simulink library "stopSim_ul"  (R2020a)
settings: Solver=VariableStepAuto  StartTime=0.0  StopTime=10.0  RelTol=1e-3
libraries: simulink x2
settings Model: Creator=John Jr  LastModifiedBy=John Jr
settings SFSimCC: CustomCodeUndefinedFunction=UseInterfaceOnly

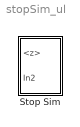
== system stopSim_ul ==
  Stop Sim : Subsystem  mask{z_0=0, t_b=0}
      mask prompts: z_0 "Initial altitude [m]"; t_b "Rocket motor burn time [s]"
      mask Display:
      | patch([0 1 1 0], [0 0 1 1],[.8 1 1])
      | 
      | port_label('input',1,'z [m]','texmode','on')
      | port_label('input',2,'t [s]','texmode','on')

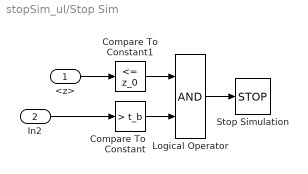
== system stopSim_ul/Stop Sim ==
  <z> : Inport
  In2 : Inport  Port=2
  Compare To Constant : simulink/Logic and Bit Operations/Compare To Constant  relop=>  const=t_b  OutDataTypeStr=boolean
  Compare To Constant1 : simulink/Logic and Bit Operations/Compare To Constant  relop=<=  const=z_0  OutDataTypeStr=boolean
  Logical Operator : Logic  AllPortsSameDT=off  OutDataTypeStr=boolean
  Stop Simulation : Stop
  wires:
  Compare To Constant1/1 -> Logical Operator/1
  Compare To Constant/1 -> Logical Operator/2
  Logical Operator/1 -> Stop Simulation/1
  In2/1 -> Compare To Constant/1
  <z>/1 -> Compare To Constant1/1
